simulink model "DLTDC1"  (R2024a)
settings: Solver=VariableStepAuto  StartTime=0.0  StopTime=50*1e-9  RelTol=1e-3
settings Model: Creator=sjtu  LastModifiedBy=sjtu

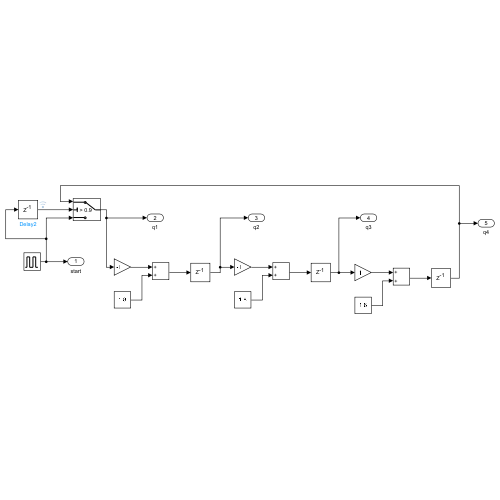
[thumbnail: Simulink's stored preview of the top-level diagram]
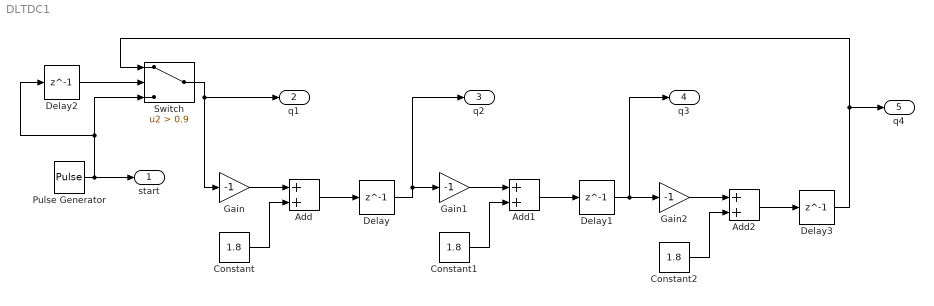
== system DLTDC1 ==
  Add : Sum
  Add1 : Sum
  Add2 : Sum
  Constant : Constant  Value=1.8
  Constant1 : Constant  Value=1.8
  Constant2 : Constant  Value=1.8
  Delay{,1..3} (4 alike) : Delay  DelayLength=1  InitialCondition=0  SampleTime=100e-12
  Gain : Gain  Gain=-1
  Gain1 : Gain  Gain=-1
  Gain2 : Gain  Gain=-1
  Pulse Generator : DiscretePulseGenerator  PulseType=Time based  Amplitude=1.8  Period=20*1e-9  PulseWidth=50  PhaseDelay=1e-9
  Switch : Switch  Criteria=u2 > Threshold  Threshold=0.9  SaturateOnIntegerOverflow=off  InputSameDT=off
  start : Outport
  q1 : Outport  Port=2
  q2 : Outport  Port=3
  q3 : Outport  Port=4
  q4 : Outport  Port=5
  wires:
  Gain/1 -> Add/1
  Constant/1 -> Add/2
  Add/1 -> Delay/1
  Constant1/1 -> Add1/2
  Add1/1 -> Delay1/1
  Gain1/1 -> Add1/1
  Delay/1 -> q2/1, Gain1/1
  Delay1/1 -> Gain2/1, q3/1
  Pulse Generator/1 -> start/1, Delay2/1, Switch/3
  Switch/1 -> q1/1, Gain/1
  Delay2/1 -> Switch/2
  Add2/1 -> Delay3/1
  Delay3/1 -> Switch/1, q4/1
  Constant2/1 -> Add2/2
  Gain2/1 -> Add2/1
